simulink model "DM_simulink"  (R2019a)
settings: Solver=FixedStepAuto  StartTime=0.0  StopTime=100  FixedStep=0.01  RelTol=1e-3
values from neighbouring files (symbols this model uses):
  Eps_p = -(eig_vals(3)+eig_vals(4))/(2*om_np)    [DM_londitudinal.m]
  Eps_sp = -(eig_vals(1)+eig_vals(2))/(2*om_nsp)    [DM_londitudinal.m]
  initial_state = [0;0;0;0]    [DM_londitudinal.m]
  om_np = sqrt(eig_vals(3)*eig_vals(4))    [DM_londitudinal.m]
  om_nsp = sqrt(eig_vals(1)*eig_vals(2))    [DM_londitudinal.m]
  theta0 = 2.2 * pi/180    (= 0.0383972435439)    [DM_londitudinal.m]    (also in main.m = 7.5)
  U0 = 94.8    [DM_londitudinal.m]    (also in main.m = 235.9)
libraries: cstblocks x2
settings Model: Creator=boiti  LastModifiedBy=boiti

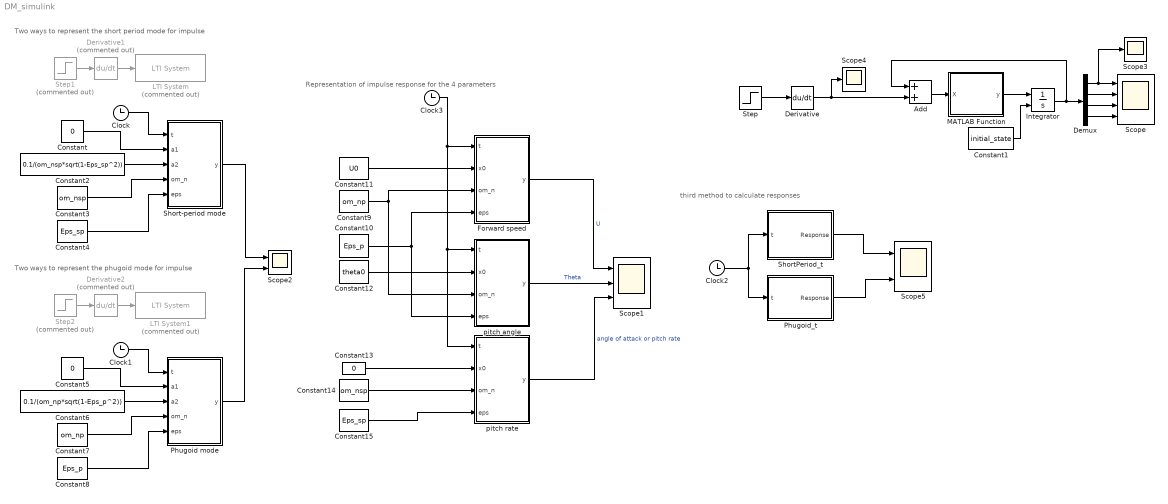
== system DM_simulink ==
  note: Representation of impulse response for the 4 parameters
  note: third method to calculate responses
  note: Two ways to represent the short period mode for impulse
  note: Two ways to represent the phugoid mode for impulse
  Add : Sum
  Clock{,1..3} (4 alike) : Clock
  Constant : Constant  Value=0
  Constant1 : Constant  Value=initial_state
  Constant10 : Constant  Value=Eps_p
  Constant11 : Constant  Value=U0
  Constant12 : Constant  Value=theta0
  Constant13 : Constant  Value=0
  Constant14 : Constant  Value=om_nsp
  Constant15 : Constant  Value=Eps_sp
  Constant2 : Constant  Value=0.1/(om_nsp*sqrt(1-Eps_sp^2))
  Constant3 : Constant  Value=om_nsp
  Constant4 : Constant  Value=Eps_sp
  Constant5 : Constant  Value=0
  Constant6 : Constant  Value=0.1/(om_np*sqrt(1-Eps_p^2))
  Constant7 : Constant  Value=om_np
  Constant8 : Constant  Value=Eps_p
  Constant9 : Constant  Value=om_np
  Demux : Demux
  Derivative : Derivative
  Derivative1 : Derivative  Commented=on
  Derivative2 : Derivative  Commented=on
  Forward speed : MATLAB Function  TreatAsAtomicUnit=on
  Integrator : Integrator  InitialConditionSource=external
  LTI System : cstblocks/LTI System  Commented=on  sys=G_sp  IC=[]
  LTI System1 : cstblocks/LTI System  Commented=on  sys=G_p  IC=[]
  MATLAB Function : MATLAB Function  TreatAsAtomicUnit=on
  Phugoid mode : MATLAB Function  TreatAsAtomicUnit=on
  Phugoid_t : MATLAB Function  TreatAsAtomicUnit=on
  Scope : Scope  NumInputPorts=4
  Scope1 : Scope  NumInputPorts=3
  Scope2 : Scope  NumInputPorts=2
  Scope3 : Scope
  Scope4 : Scope
  Scope5 : Scope  NumInputPorts=2
  Short-period mode : MATLAB Function  TreatAsAtomicUnit=on
  ShortPeriod_t : MATLAB Function  TreatAsAtomicUnit=on
  Step : Step  Time=0.01  Before=[0;0;0;0]  After=[1;0;0;0]  SampleTime=0
  Step1 : Step  Commented=on  SampleTime=0
  Step2 : Step  Commented=on  SampleTime=0
  pitch angle : MATLAB Function  TreatAsAtomicUnit=on
  pitch rate : MATLAB Function  TreatAsAtomicUnit=on
  wires:
  MATLAB Function/1(y) -> Integrator/1
  Constant1/1 -> Integrator/2
  Demux/4 -> Scope/4
  Demux/3 -> Scope/3
  Demux/2 -> Scope/2
  Demux/1 -> Scope3/1, Scope/1
  Integrator/1 -> Add/1, Demux/1
  Clock/1 -> Short-period mode/1(t)
  Constant/1 -> Short-period mode/2(a1)
  Constant2/1 -> Short-period mode/3(a2)
  Constant3/1 -> Short-period mode/4(om_n)
  Constant4/1 -> Short-period mode/5(eps)
  Short-period mode/1(y) -> Scope2/1
  Step/1 -> Derivative/1
  Derivative/1 -> Scope4/1, Add/2
  Add/1 -> MATLAB Function/1(X)
  Step1/1 -> Derivative1/1
  Derivative1/1 -> LTI System/1
  Derivative2/1 -> LTI System1/1
  Step2/1 -> Derivative2/1
  Clock1/1 -> Phugoid mode/1(t)
  Constant8/1 -> Phugoid mode/5(eps)
  Constant7/1 -> Phugoid mode/4(om_n)
  Phugoid mode/1(y) -> Scope2/2
  Constant5/1 -> Phugoid mode/2(a1)
  Constant6/1 -> Phugoid mode/3(a2)
  Phugoid_t/1(Response) -> Scope5/2
  Clock2/1 -> Phugoid_t/1(t), ShortPeriod_t/1(t)
  ShortPeriod_t/1(Response) -> Scope5/1
  Constant11/1 -> Forward speed/2(x0)
  Constant9/1 -> pitch angle/3(om_n), Forward speed/3(om_n)
  Constant10/1 -> pitch angle/4(eps), Forward speed/4(eps)
  Clock3/1 -> Forward speed/1(t), pitch rate/1(t), pitch angle/1(t)
  Constant12/1 -> pitch angle/2(x0)
  Constant13/1 -> pitch rate/2(x0)
  Constant14/1 -> pitch rate/3(om_n)
  Constant15/1 -> pitch rate/4(eps)
  pitch angle/1(y) -> Scope1/2  "Theta"
  Forward speed/1(y) -> Scope1/1  "U"
  pitch rate/1(y) -> Scope1/3  "angle of attack or pitch rate"

== matlab function DM_simulink/Short-period mode ==
  data: t input; y output; a1 input; a2 input; om_n input; eps input
function y = fcn(t, a1, a2, om_n, eps)

y = exp(-eps*om_n*t) * (a1*cos(om_n*sqrt(1-eps^2)*t) + a2*sin(om_n*sqrt(1-eps^2)*t));

== matlab function DM_simulink/MATLAB Function ==
  data: X input; y output; matrix_A parameter
function y = fcn(X, matrix_A)

y = matrix_A*X;

== matlab function DM_simulink/Phugoid mode ==
  data: t input; y output; a1 input; a2 input; om_n input; eps input
function y = fcn(t, a1, a2, om_n, eps)

y = exp(-eps*om_n*t) * (a1*cos(om_n*sqrt(1-eps^2)*t) + a2*sin(om_n*sqrt(1-eps^2)*t));

== matlab function DM_simulink/Forward speed ==
  data: t input; y output; x0 input; om_n input; eps input
function y = fcn(t, x0, om_n, eps)
a1 = x0;
a2 = (1 + a1*om_n*eps)/(om_n*sqrt(1-eps^2));
y = exp(-eps*om_n*t) * (a1*cos(om_n*sqrt(1-eps^2)*t) + a2*sin(om_n*sqrt(1-eps^2)*t));

== matlab function DM_simulink/ShortPeriod_t ==
  data: t input; Response output
function Response = ShortPeriod_t(t)
%#codegen

%    This function was generated by the Symbolic Math Toolbox version 8.3.
%    27-Apr-2020 23:00:56

t2 = 1.910922889758482e+14;
Response = t2.*exp(t.*(-3.23507389964075e-1)).*sin(t.*t2.*4.884981308350689e-15).*5.605969989267096e-15;

== matlab function DM_simulink/pitch angle ==
  data: t input; y output; x0 input; om_n input; eps input
function y = fcn(t, x0, om_n, eps)
a1 = x0;
a2 = (1 + a1*om_n*eps)/(om_n*sqrt(1-eps^2));
y = exp(-eps*om_n*t) * (a1*cos(om_n*sqrt(1-eps^2)*t) + a2*sin(om_n*sqrt(1-eps^2)*t));

== matlab function DM_simulink/Phugoid_t ==
  data: t input; Response output
function Response = Phugoid_t(t)
%#codegen

%    This function was generated by the Symbolic Math Toolbox version 8.3.
%    27-Apr-2020 23:00:59

t2 = 1.051828182895945e+16;
Response = t2.*exp(t.*(-2.491521208616993e-3)).*sin(t.*t2.*9.540979117872439e-18).*9.473652451979431e-16;

== matlab function DM_simulink/pitch rate ==
  data: t input; y output; x0 input; om_n input; eps input
function y = fcn(t, x0, om_n, eps)
a1 = x0;
a2 = (1 + a1*om_n*eps)/(om_n*sqrt(1-eps^2));
y = exp(-eps*om_n*t) * (a1*cos(om_n*sqrt(1-eps^2)*t) + a2*sin(om_n*sqrt(1-eps^2)*t));
